simulink library "Simple_EPS_lib"  (R2014a)
settings: Solver=ode45  StartTime=0.0  StopTime=10.0  RelTol=1e-3
PreLoadFcn:
  | addpath('pic')
libraries: sm_lib x7, fl_lib x4, nesl_utility x4
settings Model: Creator=ahirata  LastModifiedBy=ahirata

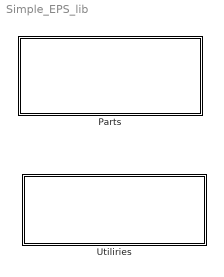
== system Simple_EPS_lib ==
  Parts : Subsystem
  Utiliries : Subsystem

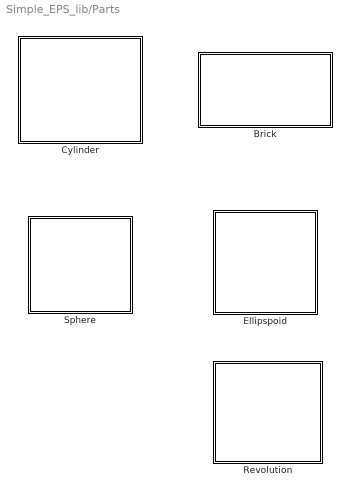
== system Simple_EPS_lib/Parts ==
  Brick : Subsystem  mask{x=300, y=50, z=50, tp=Density, In=1000, color=[1 1 0.2], con_x=None, con_y=None, con_z=None, c_p=off}
      mask prompts: x "X-axis [mm]"; y "Y-axis [mm]"; z "Z-axis [mm]"; tp "Type"; In "Density [kg/m^3] or Mass [kg]"; con_x "Connection X axis"; con_y "Connection Y axis"; con_z "Connection Z axis"; c_p "Center Position"
      mask init:
      | if tp==1
      | set_param([gcb '/Left Rack'],'DensityBased','on');
      | elseif tp==2
      | set_param([gcb '/Left Rack'],'DensityBased','off');
      | end
      | 
      | tp_ch = get_param([gcb '/Left Rack'],'DensityBased');
      | if strcmp(tp_ch,'on')==1
      |     type='Density';    
      | elseif strcmp(tp_ch,'off')==1
      |     type='Mass';
      | end
      |     
      | if con_x ==1
      |     axle_delete('-X','X_offset2')
      |     axle_delete('+X','X_offset1')
      |  elseif con_x ==2   
      |     axle_delete('-X','X_offset2')
      |     axle_add('+X','X_offset1','+','x')
      |  elseif con_x ==3
      |     axle_delete('+X','X_offset1')
      |     axle_add('-X','X_offset2','-','x')
      |  elseif con_x ==4
      |     axle_add('+X','X_offset1','+','x')
      |     axle_add('-X','X_offset2','-','x')
      | end
      | 
      | if con_y ==1
      |     axle_delete('-Y','Y_offset2')
      |     axle_delete('+Y','Y_offset1')
      |  elseif con_y ==2   
      |     axle_delete('-Y','Y_offset2')
      |     axle_add('+Y','Y_offset1','+','y')
      |  elseif con_y ==3
      |     axle_delete('+Y','Y_offset1')
      |     axle_add('-Y','Y_offset2','-','y')
      |  elseif con_y ==4
      |     axle_add('+Y','Y_offset1','+','y')
      |     axle_add('-Y','Y_offset2','-','y')
      | end
      | 
      | if con_z ==1
      |     axle_delete('-Z','Z_offset2')
      |     axle_delete('+Z','Z_offset1')
      |  elseif con_z ==2   
      |     axle_delete('-Z','Z_offset2')
      |     axle_add('+Z','Z_offset1','+','z')
      |  elseif con_z ==3
      |     axle_delete('+Z','Z_offset1')
      |     axle_add('-Z','Z_offset2','-','z')
      |  elseif con_z ==4
      |     axle_add('+Z','Z_offset1','+','z')
      |     axle_add('-Z','Z_offset2','-','z')
      | end
      | 
      | 
      | if c_p ==1
      |     axle_add('CP',[],[],[])
      | 
      | elseif c_p==0
      |     axle_delete('CP',[])
      | end
      mask TypeOptions tp: Density | Mass
      mask TypeOptions con_x: None | + direction | - direction | Both
      mask TypeOptions con_y: None | + direction | - direction | Both
      mask TypeOptions con_z: None | + direction | - direction | Both
      mask DialogControl DescGroupVar Prompt: %<MaskType>Bricks
      mask Display:
      | image('Brick.png');
      | text(0.5,0.5,type);
      | 
      | pc=get_param(gcb,'PortConnectivity');
      | blk=get_param(gcb,'Blocks');
      | 
      | b_n=size(blk,1);
      | n=size(pc,1);
      | blkl_n='';
      | blkr_n='';
      | 
      | for i=1:b_n
      | if strcmp(get_param([gcb '/' blk{i}],'BlockType'),'PMIOPort')==1 ...
      |         && strcmp(get_param([gcb '/' blk{i}],'Side'),'Left')==1
      |     blkl_n=[blkl_n; blk(i)];
      | elseif strcmp(get_param([gcb '/' blk{i}],'BlockType'),'PMIOPort')==1 ...
      |         && strcmp(get_param([gcb '/' blk{i}],'Side'),'Right')==1
      |         blkr_n=[blkr_n; blk(i)];
      | end
      | end
      | 
      | blk_n=[blkl_n; blkr_n];
      | 
      | for i=1:n
      |      pc(i).name=char(blk_n(i));
      |      port_label(pc(i).Type(1:5),str2num(pc(i).Type(6)),pc(i).name);
      | end
  Cylinder : Subsystem  mask{rd=300, lg=500, tp=Density, In=1000, color=[0 1 1], con_x=None, con_y=None, con_z=None, c_p=off}
      mask prompts: rd "Radius [mm]"; lg "Length [mm]"; tp "Type"; In "Density [kg/m^3] or Mass [kg]"; con_x "Connection X axis"; con_y "Connection Y axis"; con_z "Connection Z axis"; c_p "Center Position"
      mask init:
      | if tp==1
      | set_param([gcb '/Left Rack'],'DensityBased','on');
      | elseif tp==2
      | set_param([gcb '/Left Rack'],'DensityBased','off');
      | end
      | 
      | tp_ch = get_param([gcb '/Left Rack'],'DensityBased');
      | if strcmp(tp_ch,'on')==1
      |     type='Density';    
      | elseif strcmp(tp_ch,'off')==1
      |     type='Mass';
      | end
      |     
      | if con_x ==1
      |     axle_delete('-X','X_offset2')
      |     axle_delete('+X','X_offset1')
      |  elseif con_x ==2   
      |     axle_delete('-X','X_offset2')
      |     axle_add_c('+X','X_offset1','+','x')
      |  elseif con_x ==3
      |     axle_delete('+X','X_offset1')
      |     axle_add_c('-X','X_offset2','-','x')
      |  elseif con_x ==4
      |     axle_add_c('+X','X_offset1','+','x')
      |     axle_add_c('-X','X_offset2','-','x')
      | end
      | 
      | if con_y ==1
      |     axle_delete('-Y','Y_offset2')
      |     axle_delete('+Y','Y_offset1')
      |  elseif con_y ==2   
      |     axle_delete('-Y','Y_offset2')
      |     axle_add_c('+Y','Y_offset1','+','y')
      |  elseif con_y ==3
      |     axle_delete('+Y','Y_offset1')
      |     axle_add_c('-Y','Y_offset2','-','y')
      |  elseif con_y ==4
      |     axle_add_c('+Y','Y_offset1','+','y')
      |     axle_add_c('-Y','Y_offset2','-','y')
      | end
      | 
      | if con_z ==1
      |     axle_delete('-Z','Z_offset2')
      |     axle_delete('+Z','Z_offset1')
      |  elseif con_z ==2   
      |     axle_delete('-Z','Z_offset2')
      |     axle_add_c('+Z','Z_offset1','+','z')
      |  elseif con_z ==3
      |     axle_delete('+Z','Z_offset1')
      |     axle_add_c('-Z','Z_offset2','-','z')
      |  elseif con_z ==4
      |     axle_add_c('+Z','Z_offset1','+','z')
      |     axle_add_c('-Z','Z_offset2','-','z')
      | end
      | 
      | 
      | if c_p ==1
      |     axle_add_c('CP',[],[],[])
      | 
      | elseif c_p==0
      |     axle_delete('CP',[])
      | end
      mask TypeOptions tp: Density | Mass
      mask TypeOptions con_x: None | + direction | - direction | Both
      mask TypeOptions con_y: None | + direction | - direction | Both
      mask TypeOptions con_z: None | + direction | - direction | Both
      mask DialogControl DescGroupVar Prompt: %<MaskType>Bricks
      mask Display:
      | image('Cylinder-longitudinal.png')
      | text(0.5,0.5,type);
      | 
      | pc=get_param(gcb,'PortConnectivity');
      | blk=get_param(gcb,'Blocks');
      | 
      | b_n=size(blk,1);
      | n=size(pc,1);
      | blkl_n='';
      | blkr_n='';
      | 
      | for i=1:b_n
      | if strcmp(get_param([gcb '/' blk{i}],'BlockType'),'PMIOPort')==1 ...
      |         && strcmp(get_param([gcb '/' blk{i}],'Side'),'Left')==1
      |     blkl_n=[blkl_n; blk(i)];
      | elseif strcmp(get_param([gcb '/' blk{i}],'BlockType'),'PMIOPort')==1 ...
      |         && strcmp(get_param([gcb '/' blk{i}],'Side'),'Right')==1
      |         blkr_n=[blkr_n; blk(i)];
      | end
      | end
      | 
      | blk_n=[blkl_n; blkr_n];
      | 
      | for i=1:n
      |      pc(i).name=char(blk_n(i));
      |      port_label(pc(i).Type(1:5),str2num(pc(i).Type(6)),pc(i).name);
      | end
  Ellipspoid : Subsystem  mask{x=300, y=100, z=200, tp=Density, In=1000, color=[0 1 0], con_x=None, con_y=None, con_z=None, c_p=off}
      mask prompts: x "X-radius [mm]"; y "Y-radius [mm]"; z "Z-radius [mm]"; tp "Type"; In "Density [kg/m^3] or Mass [kg]"; con_x "Connection X axis"; con_y "Connection Y axis"; con_z "Connection Z axis"; c_p "Center Position"
      mask init:
      | if tp==1
      | set_param([gcb '/Left Rack'],'DensityBased','on');
      | elseif tp==2
      | set_param([gcb '/Left Rack'],'DensityBased','off');
      | end
      | 
      | tp_ch = get_param([gcb '/Left Rack'],'DensityBased');
      | if strcmp(tp_ch,'on')==1
      |     type='Density';    
      | elseif strcmp(tp_ch,'off')==1
      |     type='Mass';
      | end
      |     
      | if con_x ==1
      |     axle_delete('-X','X_offset2')
      |     axle_delete('+X','X_offset1')
      |  elseif con_x ==2   
      |     axle_delete('-X','X_offset2')
      |     axle_add_el('+X','X_offset1','+','x')
      |  elseif con_x ==3
      |     axle_delete('+X','X_offset1')
      |     axle_add_el('-X','X_offset2','-','x')
      |  elseif con_x ==4
      |     axle_add_el('+X','X_offset1','+','x')
      |     axle_add_el('-X','X_offset2','-','x')
      | end
      | 
      | if con_y ==1
      |     axle_delete('-Y','Y_offset2')
      |     axle_delete('+Y','Y_offset1')
      |  elseif con_y ==2   
      |     axle_delete('-Y','Y_offset2')
      |     axle_add_el('+Y','Y_offset1','+','y')
      |  elseif con_y ==3
      |     axle_delete('+Y','Y_offset1')
      |     axle_add_el('-Y','Y_offset2','-','y')
      |  elseif con_y ==4
      |     axle_add_el('+Y','Y_offset1','+','y')
      |     axle_add_el('-Y','Y_offset2','-','y')
      | end
      | 
      | if con_z ==1
      |     axle_delete('-Z','Z_offset2')
      |     axle_delete('+Z','Z_offset1')
      |  elseif con_z ==2   
      |     axle_delete('-Z','Z_offset2')
      |     axle_add_el('+Z','Z_offset1','+','z')
      |  elseif con_z ==3
      |     axle_delete('+Z','Z_offset1')
      |     axle_add_el('-Z','Z_offset2','-','z')
      |  elseif con_z ==4
      |     axle_add_el('+Z','Z_offset1','+','z')
      |     axle_add_el('-Z','Z_offset2','-','z')
      | end
      | 
      | 
      | if c_p ==1
      |     axle_add_el('CP',[],[],[])
      | 
      | elseif c_p==0
      |     axle_delete('CP',[])
      | end
      mask TypeOptions tp: Density | Mass
      mask TypeOptions con_x: None | + direction | - direction | Both
      mask TypeOptions con_y: None | + direction | - direction | Both
      mask TypeOptions con_z: None | + direction | - direction | Both
      mask DialogControl DescGroupVar Prompt: %<MaskType>Bricks
      mask Display:
      | image('Ellipsoid.png');
      | 
      | text(0.5,0.5,type);
      | 
      | pc=get_param(gcb,'PortConnectivity');
      | blk=get_param(gcb,'Blocks');
      | 
      | b_n=size(blk,1);
      | n=size(pc,1);
      | blkl_n='';
      | blkr_n='';
      | 
      | for i=1:b_n
      | if strcmp(get_param([gcb '/' blk{i}],'BlockType'),'PMIOPort')==1 ...
      |         && strcmp(get_param([gcb '/' blk{i}],'Side'),'Left')==1
      |     blkl_n=[blkl_n; blk(i)];
      | elseif strcmp(get_param([gcb '/' blk{i}],'BlockType'),'PMIOPort')==1 ...
      |         && strcmp(get_param([gcb '/' blk{i}],'Side'),'Right')==1
      |         blkr_n=[blkr_n; blk(i)];
      | end
      | end
      | 
      | blk_n=[blkl_n; blkr_n];
      | 
      | for i=1:n
      |      pc(i).name=char(blk_n(i));
      |      port_label(pc(i).Type(1:5),str2num(pc(i).Type(6)),pc(i).name);
      | end
  Revolution : Subsystem  mask{rd=50, rd_in=30, lg=100, tp=Density, In=1000, color=[1 0 0], con_x=None, con_y=None, con_z=None, c_p=off}
      mask prompts: rd "Radius [mm]"; rd_in "Bore [mm]"; lg "Lenngth [mm]"; tp "Type"; In "Density [kg/m^3] or Mass [kg]"; con_x "Connection X axis"; con_y "Connection Y axis"; con_z "Connection Z axis"; c_p "Center Position"
      mask init: same as Simple_EPS_lib/Parts/Cylinder
      mask TypeOptions tp: Density | Mass
      mask TypeOptions con_x: None | + direction | - direction | Both
      mask TypeOptions con_y: None | + direction | - direction | Both
      mask TypeOptions con_z: None | + direction | - direction | Both
      mask DialogControl DescGroupVar Prompt: %<MaskType>Bricks
      mask Display:
      | image('rote.png')
      | text(0.5,0.5,type);
      | 
      | pc=get_param(gcb,'PortConnectivity');
      | blk=get_param(gcb,'Blocks');
      | 
      | b_n=size(blk,1);
      | n=size(pc,1);
      | blkl_n='';
      | blkr_n='';
      | 
      | for i=1:b_n
      | if strcmp(get_param([gcb '/' blk{i}],'BlockType'),'PMIOPort')==1 ...
      |         && strcmp(get_param([gcb '/' blk{i}],'Side'),'Left')==1
      |     blkl_n=[blkl_n; blk(i)];
      | elseif strcmp(get_param([gcb '/' blk{i}],'BlockType'),'PMIOPort')==1 ...
      |         && strcmp(get_param([gcb '/' blk{i}],'Side'),'Right')==1
      |         blkr_n=[blkr_n; blk(i)];
      | end
      | end
      | 
      | blk_n=[blkl_n; blkr_n];
      | 
      | for i=1:n
      |      pc(i).name=char(blk_n(i));
      |      port_label(pc(i).Type(1:5),str2num(pc(i).Type(6)),pc(i).name);
      | end
  Sphere : Subsystem  mask{rd=300, tp=Density, In=1000, color=[1.0 0.4 1.0], con_x=None, con_y=None, con_z=None, c_p=off}
      mask prompts: rd "Radius [mm]"; tp "Type"; In "Density [kg/m^3] or Mass [kg]"; con_x "Connection X axis"; con_y "Connection Y axis"; con_z "Connection Z axis"; c_p "Center Position"
      mask init:
      | if tp==1
      | set_param([gcb '/Left Rack'],'DensityBased','on');
      | elseif tp==2
      | set_param([gcb '/Left Rack'],'DensityBased','off');
      | end
      | 
      | tp_ch = get_param([gcb '/Left Rack'],'DensityBased');
      | if strcmp(tp_ch,'on')==1
      |     type='Density';    
      | elseif strcmp(tp_ch,'off')==1
      |     type='Mass';
      | end
      |     
      | if con_x ==1
      |     axle_delete('-X','X_offset2')
      |     axle_delete('+X','X_offset1')
      |  elseif con_x ==2   
      |     axle_delete('-X','X_offset2')
      |     axle_add_q('+X','X_offset1','+','x')
      |  elseif con_x ==3
      |     axle_delete('+X','X_offset1')
      |     axle_add_q('-X','X_offset2','-','x')
      |  elseif con_x ==4
      |     axle_add_q('+X','X_offset1','+','x')
      |     axle_add_q('-X','X_offset2','-','x')
      | end
      | 
      | if con_y ==1
      |     axle_delete('-Y','Y_offset2')
      |     axle_delete('+Y','Y_offset1')
      |  elseif con_y ==2   
      |     axle_delete('-Y','Y_offset2')
      |     axle_add_q('+Y','Y_offset1','+','y')
      |  elseif con_y ==3
      |     axle_delete('+Y','Y_offset1')
      |     axle_add_q('-Y','Y_offset2','-','y')
      |  elseif con_y ==4
      |     axle_add_q('+Y','Y_offset1','+','y')
      |     axle_add_q('-Y','Y_offset2','-','y')
      | end
      | 
      | if con_z ==1
      |     axle_delete('-Z','Z_offset2')
      |     axle_delete('+Z','Z_offset1')
      |  elseif con_z ==2   
      |     axle_delete('-Z','Z_offset2')
      |     axle_add_q('+Z','Z_offset1','+','z')
      |  elseif con_z ==3
      |     axle_delete('+Z','Z_offset1')
      |     axle_add_q('-Z','Z_offset2','-','z')
      |  elseif con_z ==4
      |     axle_add_q('+Z','Z_offset1','+','z')
      |     axle_add_q('-Z','Z_offset2','-','z')
      | end
      | 
      | 
      | if c_p ==1
      |     axle_add_q('CP',[],[],[])
      | 
      | elseif c_p==0
      |     axle_delete('CP',[])
      | end
      mask TypeOptions tp: Density | Mass
      mask TypeOptions con_x: None | + direction | - direction | Both
      mask TypeOptions con_y: None | + direction | - direction | Both
      mask TypeOptions con_z: None | + direction | - direction | Both
      mask DialogControl DescGroupVar Prompt: %<MaskType>Bricks
      mask Display:
      | image('Sphere.png')
      | 
      | text(0.5,0.5,type);
      | 
      | pc=get_param(gcb,'PortConnectivity');
      | blk=get_param(gcb,'Blocks');
      | 
      | b_n=size(blk,1);
      | n=size(pc,1);
      | blkl_n='';
      | blkr_n='';
      | 
      | for i=1:b_n
      | if strcmp(get_param([gcb '/' blk{i}],'BlockType'),'PMIOPort')==1 ...
      |         && strcmp(get_param([gcb '/' blk{i}],'Side'),'Left')==1
      |     blkl_n=[blkl_n; blk(i)];
      | elseif strcmp(get_param([gcb '/' blk{i}],'BlockType'),'PMIOPort')==1 ...
      |         && strcmp(get_param([gcb '/' blk{i}],'Side'),'Right')==1
      |         blkr_n=[blkr_n; blk(i)];
      | end
      | end
      | 
      | blk_n=[blkl_n; blkr_n];
      | 
      | for i=1:n
      |      pc(i).name=char(blk_n(i));
      |      port_label(pc(i).Type(1:5),str2num(pc(i).Type(6)),pc(i).name);
      | end

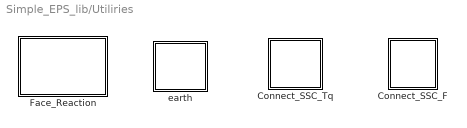
== system Simple_EPS_lib/Utiliries ==
  Connect_SSC_F : Subsystem
  Connect_SSC_Tq : Subsystem
  Face_Reaction : Subsystem  mask{Kp=100000, Kd=10000, add=off}
      mask prompts: Kp "Kp_gain"; Kd "Kd_gain"; add "Add Force"
      mask init:
      | load_system('simulink')
      | 
      | msk_blk = get_param(gcb,'Blocks');
      | ck = sum(strcmp(msk_blk,'add'));
      | if add == 1 && ck==0
      |     delete_line(gcb,'Cons_zero/1','Sum1/1')
      |     delete_block([gcb '/Cons_zero'])
      | 
      |     add_block('simulink/Sources/In1', [gcb '/add'])
      |     add_line(gcb,'add/1','Sum1/1')
      | 
      |     
      | elseif add == 0 && ck ==1
      |         delete_line(gcb,'add/1','Sum1/1')
      |         delete_block([gcb '/add'])
      |         
      |         add_block('simulink/Sources/Constant', [gcb '/Cons_zero'],'Value','0')
      |         add_line(gcb,'Cons_zero/1','Sum1/1')
      |   
      | end
      mask Display:
      | image('ground.png')
      | port_label('LConn', 1, 'Velocity')
      | port_label('LConn', 2, 'Position')
      | port_label('RConn', 1, 'Re_f')
  earth : Subsystem
      mask Display: image('earth.png')

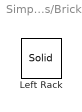
== system Simple_EPS_lib/Parts/Brick ==
  Left Rack : sm_lib/Body Elements/Solid  InertiaType=CalculateFromGeometry  Mass=In  MassUnits=kg  CenterOfMass=[0 0 0]  CenterOfMassUnits=m  MomentsOfInertia=[1 1 1]  MomentsOfInertiaUnits=kg*m^2  ProductsOfInertia=[0 0 0]  ProductsOfInertiaUnits=kg*m^2  DensityBased=on  Density=In  DensityUnits=kg/(m^3)  GraphicType=FromGeometry  MarkerShape=Sphere  MarkerSize=10  MarkerSizeUnits=m  GraphicVisPropType=SimpleVisualProperties  GraphicDiffuseColor=color  GraphicSpecularColor=[0.5 0.5 0.5 1.0]  GraphicAmbientColor=[0.15 0.15 0.15 1.0]  GraphicEmissiveColor=[0.0 0.0 0.0 1.0]  GraphicShininess=75  GraphicOpacity=1.0  GeometryShape=Brick  RectangleSize=[1 1]  RectangleSizeUnits=m  BrickDimensions=[x y z]  BrickDimensionUnits=mm  CylinderRadius=1  CylinderRadiusUnits=m  CylinderLength=1  CylinderLengthUnits=m  SphereRadius=1  SphereRadiusUnits=m  EllipsoidRadii=[1 1 1]  EllipsoidRadiiUnits=m  ExtrusionCrossSection=0  ExtrusionCrossSectionUnits=cm  ExtrusionLength=0  ExtrusionLengthUnits=cm  PolygonNumSides=3  PolygonOuterRadius=1  PolygonOuterRadiusUnits=m  ExtGeomFileType=STL  ExtGeomFileUnits=m  RevolutionCrossSection=[1 1; 1 -1; 2 -1; 2 1]  RevolutionCrossSectionUnits=m  RevolutionExtent=Full  RevolutionAngle=180  RevolutionAngleUnits=deg  BlockFunction=simmechanics.library.body_elements.solid

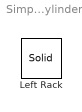
== system Simple_EPS_lib/Parts/Cylinder ==
  Left Rack : sm_lib/Body Elements/Solid  InertiaType=CalculateFromGeometry  Mass=In  MassUnits=kg  CenterOfMass=[0 0 0]  CenterOfMassUnits=m  MomentsOfInertia=[1 1 1]  MomentsOfInertiaUnits=kg*m^2  ProductsOfInertia=[0 0 0]  ProductsOfInertiaUnits=kg*m^2  DensityBased=on  Density=In  DensityUnits=kg/(m^3)  GraphicType=FromGeometry  MarkerShape=Sphere  MarkerSize=10  MarkerSizeUnits=m  GraphicVisPropType=SimpleVisualProperties  GraphicDiffuseColor=color  GraphicSpecularColor=[0.5 0.5 0.5 1.0]  GraphicAmbientColor=[0.15 0.15 0.15 1.0]  GraphicEmissiveColor=[0.0 0.0 0.0 1.0]  GraphicShininess=75  GraphicOpacity=1.0  GeometryShape=Cylinder  RectangleSize=[1 1]  RectangleSizeUnits=m  BrickDimensions=[0 0 0]  BrickDimensionUnits=mm  CylinderRadius=rd  CylinderRadiusUnits=mm  CylinderLength=lg  CylinderLengthUnits=mm  SphereRadius=1  SphereRadiusUnits=m  EllipsoidRadii=[1 1 1]  EllipsoidRadiiUnits=m  ExtrusionCrossSection=0  ExtrusionCrossSectionUnits=cm  ExtrusionLength=0  ExtrusionLengthUnits=cm  PolygonNumSides=3  PolygonOuterRadius=1  PolygonOuterRadiusUnits=m  ExtGeomFileType=STL  ExtGeomFileUnits=m  RevolutionCrossSection=[1 1; 1 -1; 2 -1; 2 1]  RevolutionCrossSectionUnits=m  RevolutionExtent=Full  RevolutionAngle=180  RevolutionAngleUnits=deg  BlockFunction=simmechanics.library.body_elements.solid

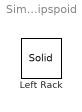
== system Simple_EPS_lib/Parts/Ellipspoid ==
  Left Rack : sm_lib/Body Elements/Solid  InertiaType=CalculateFromGeometry  Mass=In  MassUnits=kg  CenterOfMass=[0 0 0]  CenterOfMassUnits=m  MomentsOfInertia=[1 1 1]  MomentsOfInertiaUnits=kg*m^2  ProductsOfInertia=[0 0 0]  ProductsOfInertiaUnits=kg*m^2  DensityBased=on  Density=In  DensityUnits=kg/(m^3)  GraphicType=FromGeometry  MarkerShape=Sphere  MarkerSize=10  MarkerSizeUnits=m  GraphicVisPropType=SimpleVisualProperties  GraphicDiffuseColor=color  GraphicSpecularColor=[0.5 0.5 0.5 1.0]  GraphicAmbientColor=[0.15 0.15 0.15 1.0]  GraphicEmissiveColor=[0.0 0.0 0.0 1.0]  GraphicShininess=75  GraphicOpacity=1.0  GeometryShape=Ellipsoid  RectangleSize=[1 1]  RectangleSizeUnits=m  BrickDimensions=[1 1 1]  BrickDimensionUnits=mm  CylinderRadius=1  CylinderRadiusUnits=m  CylinderLength=1  CylinderLengthUnits=m  SphereRadius=1  SphereRadiusUnits=m  EllipsoidRadii=[x y z]  EllipsoidRadiiUnits=mm  ExtrusionCrossSection=0  ExtrusionCrossSectionUnits=cm  ExtrusionLength=0  ExtrusionLengthUnits=cm  PolygonNumSides=3  PolygonOuterRadius=1  PolygonOuterRadiusUnits=m  ExtGeomFileType=STL  ExtGeomFileUnits=m  RevolutionCrossSection=[1 1; 1 -1; 2 -1; 2 1]  RevolutionCrossSectionUnits=m  RevolutionExtent=Full  RevolutionAngle=180  RevolutionAngleUnits=deg  BlockFunction=simmechanics.library.body_elements.solid

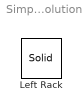
== system Simple_EPS_lib/Parts/Revolution ==
  Left Rack : sm_lib/Body Elements/Solid  InertiaType=CalculateFromGeometry  Mass=In  MassUnits=kg  CenterOfMass=[0 0 0]  CenterOfMassUnits=m  MomentsOfInertia=[1 1 1]  MomentsOfInertiaUnits=kg*m^2  ProductsOfInertia=[0 0 0]  ProductsOfInertiaUnits=kg*m^2  DensityBased=on  Density=In  DensityUnits=kg/m^3  GraphicType=FromGeometry  MarkerShape=Sphere  MarkerSize=10  MarkerSizeUnits=m  GraphicVisPropType=SimpleVisualProperties  GraphicDiffuseColor=color  GraphicSpecularColor=[0.5 0.5 0.5 1.0]  GraphicAmbientColor=[0.15 0.15 0.15 1.0]  GraphicEmissiveColor=[0.0 0.0 0.0 1.0]  GraphicShininess=75  GraphicOpacity=1.0  GeometryShape=GeneralSolidOfRevolution  RectangleSize=[1 1]  RectangleSizeUnits=m  BrickDimensions=[1 1 1]  BrickDimensionUnits=mm  CylinderRadius=1  CylinderRadiusUnits=m  CylinderLength=1  CylinderLengthUnits=m  SphereRadius=1  SphereRadiusUnits=m  EllipsoidRadii=[1 1 1]  EllipsoidRadiiUnits=mm  ExtrusionCrossSection=0  ExtrusionCrossSectionUnits=cm  ExtrusionLength=0  ExtrusionLengthUnits=mm  PolygonNumSides=0  PolygonOuterRadius=0  PolygonOuterRadiusUnits=mm  ExtGeomFileType=STL  ExtGeomFileUnits=m  RevolutionCrossSection=[rd_in lg/2; rd_in -lg/2; rd -lg/2; rd lg/2;]  RevolutionCrossSectionUnits=mm  RevolutionExtent=Full  RevolutionAngle=180  RevolutionAngleUnits=deg  BlockFunction=simmechanics.library.body_elements.solid

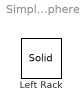
== system Simple_EPS_lib/Parts/Sphere ==
  Left Rack : sm_lib/Body Elements/Solid  InertiaType=CalculateFromGeometry  Mass=In  MassUnits=kg  CenterOfMass=[0 0 0]  CenterOfMassUnits=m  MomentsOfInertia=[1 1 1]  MomentsOfInertiaUnits=kg*m^2  ProductsOfInertia=[0 0 0]  ProductsOfInertiaUnits=kg*m^2  DensityBased=on  Density=In  DensityUnits=kg/(m^3)  GraphicType=FromGeometry  MarkerShape=Sphere  MarkerSize=10  MarkerSizeUnits=m  GraphicVisPropType=SimpleVisualProperties  GraphicDiffuseColor=color  GraphicSpecularColor=[0.5 0.5 0.5 1.0]  GraphicAmbientColor=[0.15 0.15 0.15 1.0]  GraphicEmissiveColor=[0.0 0.0 0.0 1.0]  GraphicShininess=75  GraphicOpacity=1.0  GeometryShape=Sphere  RectangleSize=[1 1]  RectangleSizeUnits=m  BrickDimensions=[1 1 1]  BrickDimensionUnits=mm  CylinderRadius=1  CylinderRadiusUnits=m  CylinderLength=1  CylinderLengthUnits=m  SphereRadius=rd  SphereRadiusUnits=mm  EllipsoidRadii=[1 1 1]  EllipsoidRadiiUnits=m  ExtrusionCrossSection=0  ExtrusionCrossSectionUnits=cm  ExtrusionLength=0  ExtrusionLengthUnits=cm  PolygonNumSides=3  PolygonOuterRadius=1  PolygonOuterRadiusUnits=m  ExtGeomFileType=STL  ExtGeomFileUnits=m  RevolutionCrossSection=[1 1; 1 -1; 2 -1; 2 1]  RevolutionCrossSectionUnits=m  RevolutionExtent=Full  RevolutionAngle=180  RevolutionAngleUnits=deg  BlockFunction=simmechanics.library.body_elements.solid

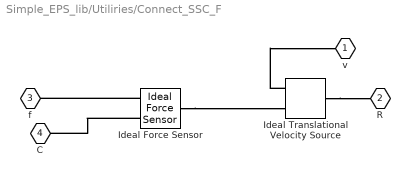
== system Simple_EPS_lib/Utiliries/Connect_SSC_F ==
  Ideal Force Sensor : fl_lib/Mechanical/Mechanical Sensors/Ideal Force Sensor
  Ideal Translational Velocity Source : fl_lib/Mechanical/Mechanical Sources/Ideal Translational Velocity Source
  v : PMIOPort  Port=1  Side=Right
  R : PMIOPort  Port=2  Side=Right
  f : PMIOPort  Port=3  Side=Left
  C : PMIOPort  Port=4  Side=Left
  connections:
  Ideal Translational Velocity Source/RConn1 -- v/RConn1
  Ideal Translational Velocity Source/LConn1 -- R/RConn1
  Ideal Force Sensor/RConn1 -- C/RConn1
  Ideal Force Sensor/RConn2 -- f/RConn1
  Ideal Force Sensor/LConn1 -- Ideal Translational Velocity Source/RConn2

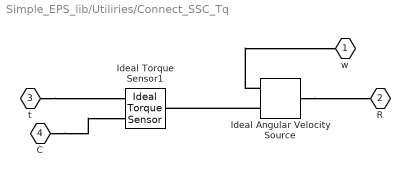
== system Simple_EPS_lib/Utiliries/Connect_SSC_Tq ==
  Ideal Angular Velocity Source : fl_lib/Mechanical/Mechanical Sources/Ideal Angular Velocity Source
  Ideal Torque Sensor1 : fl_lib/Mechanical/Mechanical Sensors/Ideal Torque Sensor
  w : PMIOPort  Port=1  Side=Right
  R : PMIOPort  Port=2  Side=Right
  t : PMIOPort  Port=3  Side=Left
  C : PMIOPort  Port=4  Side=Left
  connections:
  t/RConn1 -- Ideal Torque Sensor1/RConn2
  Ideal Angular Velocity Source/RConn2 -- Ideal Torque Sensor1/LConn1
  C/RConn1 -- Ideal Torque Sensor1/RConn1
  Ideal Angular Velocity Source/LConn1 -- R/RConn1
  Ideal Angular Velocity Source/RConn1 -- w/RConn1

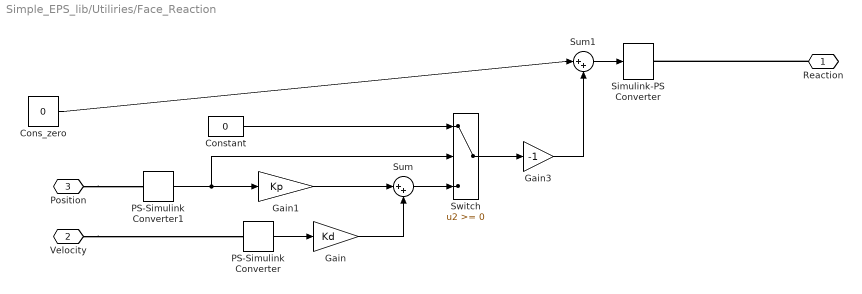
== system Simple_EPS_lib/Utiliries/Face_Reaction ==
  Cons_zero : Constant  Value=0
  Constant : Constant  Value=0
  Gain : Gain  Gain=Kd
  Gain1 : Gain  Gain=Kp
  Gain3 : Gain  Gain=-1
  PS-Simulink Converter : nesl_utility/PS-Simulink Converter  PhysicalDomain=network_engine_domain  SubClassName=ps_output  LeftPortType=input  RightPortType=output  PseudoPeriodic=off  Frequencies=[]  Unit=1  AffineConversion=off
  PS-Simulink Converter1 : nesl_utility/PS-Simulink Converter  PhysicalDomain=network_engine_domain  SubClassName=ps_output  LeftPortType=input  RightPortType=output  PseudoPeriodic=off  Frequencies=[]  Unit=1  AffineConversion=off
  Simulink-PS Converter : nesl_utility/Simulink-PS Converter  PhysicalDomain=network_engine_domain  SubClassName=ps_input  LeftPortType=input  RightPortType=output  PseudoPeriodic=off  Frequencies=[]  NoiseDistribution=none  NoiseParameters=[]  Unit=1  AffineConversion=off  InputFiltering=off  SimscapeFilterOrder=1  InputFilterTimeConstant=0.001  UdotUserProvided=1
  Sum : Sum  Inputs=|++
  Sum1 : Sum  Inputs=|++
  Switch : Switch
  Reaction : PMIOPort  Port=1  Side=Right
  Velocity : PMIOPort  Port=2  Side=Left
  Position : PMIOPort  Port=3  Side=Left
  wires:
  Cons_zero/1 -> Sum1/1
  Sum1/1 -> Simulink-PS Converter/1
  PS-Simulink Converter/1 -> Gain/1
  Gain1/1 -> Sum/1
  Gain/1 -> Sum/2
  Constant/1 -> Switch/1
  PS-Simulink Converter1/1 -> Switch/2, Gain1/1
  Switch/1 -> Gain3/1
  Sum/1 -> Switch/3
  Gain3/1 -> Sum1/2
  connections:
  Position/RConn1 -- PS-Simulink Converter1/LConn1
  Velocity/RConn1 -- PS-Simulink Converter/LConn1
  Reaction/RConn1 -- Simulink-PS Converter/RConn1

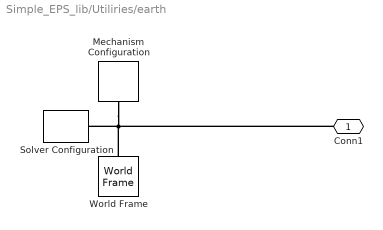
== system Simple_EPS_lib/Utiliries/earth ==
  Mechanism Configuration : sm_lib/Utilities/Mechanism Configuration  UniformGravity=Constant  GravityVector=[0 0 -9.80665]  GravityUnits=m/s^2  LinearizationDelta=0.001  BlockFunction=simmechanics.library.utilities.mechanism_configuration
  Solver Configuration : nesl_utility/Solver Configuration  PhysicalDomain=network_engine_domain  SubClassName=solver  LeftPortType=input  RightPortType=generic  Accelerate=off  Tones=[]  Harmonics=[]  SimulateNoise=off  Profile=off  UseLocalSampling=off  EnableSwitchedLinearOptims=on  FrequencyDomain=off  UseCCode=off  RelTol=0.001  AbsTol=1e-06  MinStep=1e-09  ToWorkspace=off  DoDC=off  ResidualTolerance=1e-09  UseLocalSolver=off  LocalSolverChoice=NE_BACKWARD_EULER_ADVANCER  LocalSolverSampleTime=0.001  DoFixedCost=off  MaxNonlinIter=3  MaxModeIter=2  LinearAlgebra=Sparse  DelaysMemoryBudget=1024  AutomaticFiltering=on  FilteringTimeConstant=0.001
  World Frame : sm_lib/Frames and Transforms/World Frame  BlockFunction=simmechanics.library.frames_transforms.world_frame
  Conn1 : PMIOPort  Port=1  Side=Right
  connections:
  Conn1/RConn1 -- Mechanism Configuration/RConn1 -- World Frame/RConn1 -- Solver Configuration/RConn1
